simulink library "alpha_beta_to_dq"  (R2026a)
settings: Solver=VariableStepAuto
settings Model: Creator=dbagn  LastModifiedBy=dbagn

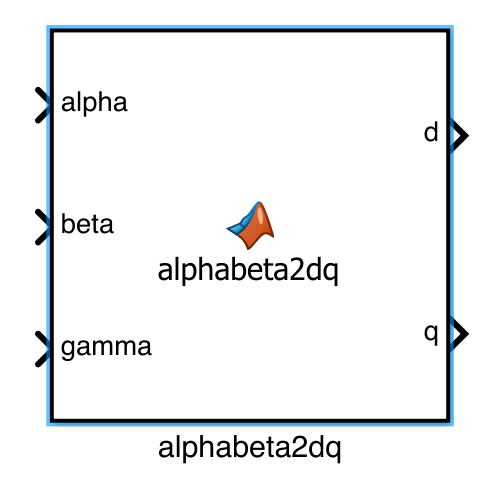
[thumbnail: Simulink's stored preview of the top-level diagram]
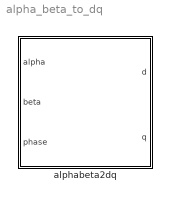
== system alpha_beta_to_dq ==
  alphabeta2dq : MATLAB Function  TreatAsAtomicUnit=on

== matlab function alpha_beta_to_dq/alphabeta2dq ==
  data: alpha input; d output; beta input; phase input; q output
function [d,q] = alphabeta2dq(alpha,beta,phase)

    d  =  alpha*cos(phase) + beta*sin(phase);
    q = -alpha*sin(phase) + beta*cos(phase);

end
